simulink model "gm_uz_mpc_3ph"  (R2021a)
settings: Solver=FixedStepDiscrete  StartTime=0.0  StopTime=2000*t_ADC  RelTol=1e-3
undefined symbols (not defined in the file or in its folder): IB, id_ref, iq_ref, lambda_d, lambda_q, lambda_u, Ld_over_LB, Lq_over_LB, n_rpm, omegaB, p, psi_pm_over_psiB, Rs_over_ZB, t_ADC, t_clock, Ts_times_ZB_over_Ld, Ts_times_ZB_over_Lq, v_dc, VB
libraries: nesl_utility x19, simulink x18, fl_lib x15, ee_lib x7, hdlsllib x2, spsAlphaBetaZerotodq0Lib x1
(part 1 of 3)
settings Model: Creator=micha  LastModifiedBy=micha
settings SolverCC: AlgebraicLoopSolver=TrustRegion
settings DataIOCC: LimitDataPoints=on  SaveOutput=off  SaveTime=off
settings OptimizationCC: BlockReduction=off  ConditionallyExecuteInputs=off  DefaultParameterBehavior=Inlined  LifeSpan=inf
settings DebuggingCC: AlgebraicLoopMsg=error  InheritedTsInSrcMsg=none  SingleTaskRateTransMsg=error  AllowSymbolicDim=off  StrictBusMsg=ErrorOnBusTreatedAsVector  SFUnexpectedBacktrackingDiag=warning  SFNoUnconditionalDefaultTransitionDiag=warning  SFExecutionAtInitializationDiag=none  SFMachineParentedDataDiag=warning  ArithmeticOperatorsInVariantConditions=warning
settings HardwareCC: ProdBitPerPointer=32  ProdBitPerSizeT=32  ProdBitPerPtrDiffT=32  ProdLargestAtomicFloat=None  ProdIntDivRoundTo=Undefined  ProdEndianess=Unspecified  ProdWordSize=32  ProdHWDeviceType=ASIC/FPGA->ASIC/FPGA  ProdEqTarget=off
settings SFSimCC: SimUseLocalCustomCode=off  CustomCodeUndefinedFunction=UseInterfaceOnly
settings RTWCC: RTWUseLocalCustomCode=off
settings CodeAppCC: StateflowObjectComments=on
settings GRTTargetCC: TargetLangStandard=C89/C90 (ANSI)
settings ConfigComp: CovScope=ReferencedModels  CovMetricSettings=dw  CovSaveCumulativeToWorkspaceVar=on  CovSaveSingleToWorkspaceVar=on  CovExternalEMLEnable=off  CovSFcnEnable=off

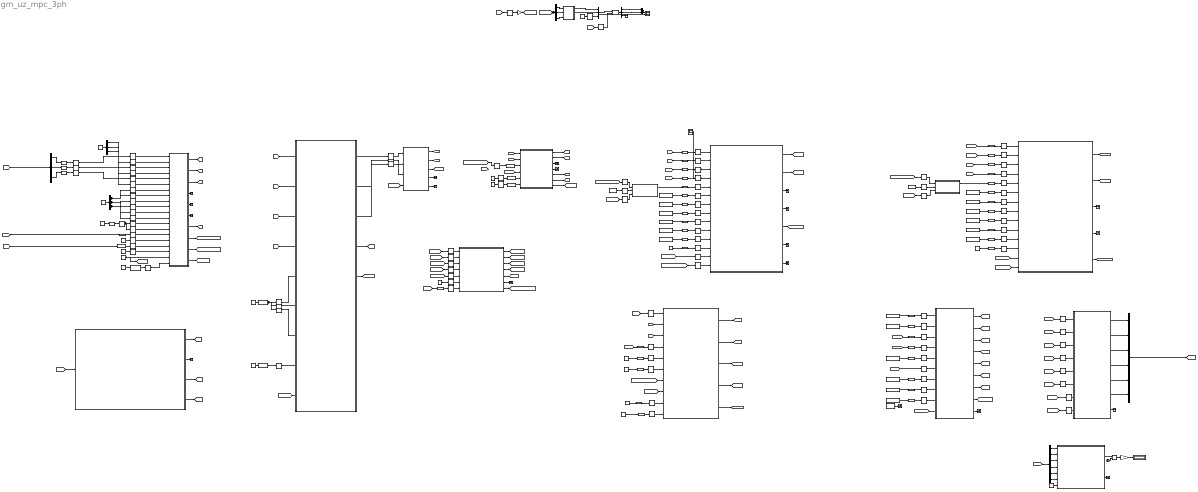
== system gm_uz_mpc_3ph ==
  note: 0=AXI 1=PL
  note: 1=real 0=debug
  note: delay compensation
  note: dynamic voltage LUT
  note: prediction model
  note: cost function
  note: gates enable
  note: average switching frequency calculation
  note: per unit conversion
  note: MPC state machine
  note: Clarke and Park transformation
  note: debug ip for input of constant measurement values
  note: inverter and motor
  Alpha-Beta-Zero to dq1 : spsAlphaBetaZerotodq0Lib/Alpha-Beta-Zero to dq0  Alignment=Aligned with phase A axis
      settings: SourceProductBaseCode=PS
  Clock : Clock
  Constant : Constant  Value=8  OutDataTypeStr=uint32  SampleTime=-1
  Constant1 : Constant  Value=p
  Constant10 : Constant  Value=psi_pm_over_psiB
  Constant{2,11,25,62} (4 alike) : Constant
  Constant12 : Constant  Value=0
  Constant13 : Constant  Value=p
  Constant14 : Constant  Value=psi_pm_over_psiB
  Constant15 : Constant  Value=Rs_over_ZB
  Constant17 : Constant  Value=Ts_times_ZB_over_Ld
  Constant18 : Constant  Value=Ts_times_ZB_over_Lq
  Constant21 : Constant  Value=Ld_over_LB
  Constant22 : Constant  Value=Lq_over_LB
  Constant26 : Constant  Value=v_dc
  Constant27 : Constant  Value=iq_ref/IB
  Constant3 : Constant  Value=Rs_over_ZB
  Constant30 : Constant  Value=0  OutDataTypeStr=uint32  SampleTime=-1
  Constant31 : Constant  Value=lambda_d
  Constant32 : Constant  Value=lambda_q
  Constant35 : Constant  Value=lambda_u
  Constant4 : Constant  Value=Ts_times_ZB_over_Ld
  Constant42 : Constant  Value=id_ref/IB
  Constant44 : Constant  Value=0.00008  SampleTime=-1
  Constant5 : Constant  Value=Ts_times_ZB_over_Lq
  Constant52 : Constant  Value=0
  Constant53 : Constant  Value=1/omegaB  OutDataTypeStr=fixdt(0,18,18)
  Constant54 : Constant  Value=1/omegaB  OutDataTypeStr=fixdt(0,18,18)
  Constant55 : Constant  Value=0  OutDataTypeStr=fixdt(1,24,11)  SampleTime=-1
  Constant56 : Constant  Value=1/IB
  Constant57 : Constant  Value=1/VB
  Constant58 : Constant  Value=63
  Constant59 : Constant  OutDataTypeStr=boolean  SampleTime=-1
  Constant6 : Constant  Value=[0 0 0]  OutDataTypeStr=fixdt(1,27,15)  SampleTime=-1
  Constant60 : Constant  Value=[1 2 3]  OutDataTypeStr=fixdt(1,27,15)  SampleTime=-1
  Constant61 : Constant  Value=0  OutDataTypeStr=fixdt(1,27,20)  SampleTime=-1
  Constant63 : Constant  Value=0.15
  Constant8 : Constant  Value=Ld_over_LB
  Constant9 : Constant  Value=Lq_over_LB
  Data Type Conversion1 : DataTypeConversion  OutDataTypeStr=boolean
  Data Type Conversion{2,6,10..11,13,65..66} (7 alike) : DataTypeConversion  OutDataTypeStr=fixdt_type_polepairs
  Data Type Conversion{12,14..15,18..22,25..28} (12 alike) : DataTypeConversion  OutDataTypeStr=fixdt_type_constants
  Data Type Conversion29 : DataTypeConversion  OutDataTypeStr=fixdt_type_speed
  Data Type Conversion30 : DataTypeConversion  OutDataTypeStr=fixdt_type_speed
  Data Type Conversion32 : DataTypeConversion  OutDataTypeStr=fixdt(0,18,18)
  Data Type Conversion33 : DataTypeConversion  OutDataTypeStr=fixdt(0,18,18)
  Data Type Conversion{34..36,68} (4 alike) : DataTypeConversion  OutDataTypeStr=fixdt(1,27,15)
  Data Type Conversion37 : DataTypeConversion  OutDataTypeStr=fixdt(1,27,20)
  Data Type Conversion39 : DataTypeConversion  OutDataTypeStr=fixdt(1,18,14)
  Data Type Conversion{4..5,44..45,52..53} (6 alike) : DataTypeConversion  OutDataTypeStr=fixdt_type_dq_currents
  Data Type Conversion{7..8,48..49} (4 alike) : DataTypeConversion  OutDataTypeStr=fixdt_type_dqxy_voltages
  Data Type Conversion54 : DataTypeConversion  OutDataTypeStr=fixdt_type_max_current
  Data Type Conversion57 : DataTypeConversion  OutDataTypeStr=fixdt_type_xy_currents
  Data Type Conversion58 : DataTypeConversion  OutDataTypeStr=fixdt_type_xy_currents
  Data Type Conversion59 : DataTypeConversion  OutDataTypeStr=fixdt(1,18,14)
  Data Type Conversion60 : DataTypeConversion  OutDataTypeStr=fixdt_type_lambda
  Data Type Conversion61 : DataTypeConversion  OutDataTypeStr=fixdt_type_lambda
  Data Type Conversion64 : DataTypeConversion  OutDataTypeStr=fixdt_type_lambda
  Data Type Conversion69 : DataTypeConversion  OutDataTypeStr=fixdt(1,24,11)
  Data Type Conversion70 : DataTypeConversion  OutDataTypeStr=fixdt(1,18,15)
  Data Type Conversion9 : DataTypeConversion  OutDataTypeStr=fixdt(1,27,20)
  Demux{,1,4..6} (5 alike) : Demux  Outputs=3
  Demux2 : Demux  Outputs=6
  Display : Display
  Divide : Product  Inputs=*/
  Gain : Gain  Gain=1/IB
  Gain19 : Gain  Gain=1/(6*2)
  Mux : Mux  Inputs=2
  Mux2 : Mux  Inputs=6
  Mux5 : Mux  Inputs=3
  Pulse Generator2 : DiscretePulseGenerator  PulseType=Time based  Period=t_ADC  PulseWidth=5
  Rate Transition : RateTransition  OutPortSampleTime=t_ADC
  Rate Transition{1..4,6..7,9..10,12..13,15,17..21,23,25,28..33,35,38..43,45..46,50,53..54,57..58,60..62,65..67,69..70,73..74,77..82,85..86,91..96,100..107,111..128,130} (89 alike) : RateTransition  OutPortSampleTime=t_clock
  Rate Transition{11,55,68,75..76,129} (6 alike) : RateTransition  InitialCondition=1  OutPortSampleTime=t_clock
  Rate Transition131 : RateTransition  OutPortSampleTime=t_ADC
  Rate Transition132 : RateTransition  OutPortSampleTime=t_ADC
  Scope : Scope  NumInputPorts=2
  Scope3 : Scope  NumInputPorts=2
  Terminator{,2..3,8..14,17..20,23..28} (20 alike) : Terminator
  clarke : MATLAB Function  TreatAsAtomicUnit=on
  cost_opt : Subsystem  TreatAsAtomicUnit=on
  counter_f_sw_3ph : Subsystem  TreatAsAtomicUnit=on
  ctrl_state_machine : Subsystem  TreatAsAtomicUnit=on
  delay_comp : Subsystem  TreatAsAtomicUnit=on
  inverter_machine : Subsystem
  mpc_enable : Subsystem  TreatAsAtomicUnit=on
  prediction : Subsystem  TreatAsAtomicUnit=on
  pu_omega_m : Subsystem  TreatAsAtomicUnit=on
  pu_omega_m1 : Subsystem
  pu_voltages_vsd : Subsystem  TreatAsAtomicUnit=on
  uz_clarke : Subsystem  TreatAsAtomicUnit=on
  uz_debug_switch_measurements : Subsystem  TreatAsAtomicUnit=on
  uz_park_transformation : Subsystem  TreatAsAtomicUnit=on
  uz_pu_conversion : Subsystem  TreatAsAtomicUnit=on
  wires:
  Demux1/3 -> Rate Transition121/1, Rate Transition122/1
  Demux1/2 -> Rate Transition120/1, Rate Transition119/1
  Demux1/1 -> Rate Transition117/1, Rate Transition118/1
  Constant6/1 -> Demux1/1
  Constant44/1 -> Terminator/1
  uz_pu_conversion/4(out3) -> [v_dc_pu]
  uz_debug_switch_measurements/6(out5) -> Terminator28/1
  uz_debug_switch_measurements/5(out4) -> Terminator27/1
  uz_debug_switch_measurements/4(out3) -> Terminator26/1
  [debug_ip_done] -> uz_pu_conversion/9(adc_valid_trigger)
  uz_debug_switch_measurements/10(debug_ip_done) -> [debug_ip_done]
  [v_dc] -> uz_pu_conversion/4(in3)
  [i_c1] -> uz_pu_conversion/3(in2)
  [i_b1] -> uz_pu_conversion/2(in1)
  [i_a1] -> uz_pu_conversion/1(in0)
  uz_debug_switch_measurements/3(out2) -> [i_c1]
  uz_debug_switch_measurements/7(out6) -> [v_dc]
  uz_debug_switch_measurements/2(out1) -> [i_b1]
  uz_debug_switch_measurements/1(out0) -> [i_a1]
  Mux/1 -> Scope/1
  Rate Transition132/1 -> Alpha-Beta-Zero to dq1/2
  Rate Transition131/1 -> Mux5/3
  Demux4/2 -> Mux/2  "iq"
  Demux4/1 -> Mux/1  "id"
  Rate Transition/1 -> Gain/1
  [pu_conv_valid] -> uz_clarke/4(pu_conv_valid)
  mpc_enable/7(enb_mpc_done) -> Terminator23/1
  [G1] -> Rate Transition96/1
  [G2] -> Rate Transition93/1
  [G3] -> Rate Transition94/1
  [G4] -> Rate Transition91/1
  [G5] -> Rate Transition92/1
  cost_opt/3(G1) -> [G1]
  cost_opt/4(G2) -> [G2]
  cost_opt/5(G3) -> [G3]
  cost_opt/6(G4) -> [G4]
  cost_opt/7(G5) -> [G5]
  [G0] -> Rate Transition95/1
  cost_opt/2(G0) -> [G0]
  prediction/4(iq_pred_pu_AXI) -> Terminator20/1
  prediction/3(id_pred_pu_AXI) -> Terminator19/1
  delay_comp/6(Rs_over_ZB) -> Terminator17/1
  delay_comp/7(Ts_times_ZB_over_Ld) -> Terminator18/1
  delay_comp/4(iq_delay_pu_AXI) -> Terminator14/1
  delay_comp/3(id_delay_pu_AXI) -> Terminator13/1
  ctrl_state_machine/6(trigger_state_machine_finished) -> Terminator12/1
  ctrl_state_machine/4(trigger_optimization) -> [trigger_optimization]
  [trigger_optimization] -> cost_opt/10(trigger_optimization)
  ctrl_state_machine/3(trigger_prediction) -> [trigger_prediciton]
  [trigger_prediciton] -> prediction/13(trigger_prediction)
  ctrl_state_machine/2(trigger_delay_comp) -> [trigger_delay_comp]
  [trigger_delay_comp] -> Rate Transition7/1
  uz_clarke/3(clarke_done) -> [clarke_done]
  [clarke_done] -> uz_park_transformation/4(trigger)
  [beta] -> uz_park_transformation/2(u2)
  [alpha] -> uz_park_transformation/1(u1)
  uz_clarke/1(alpha) -> [alpha]
  uz_clarke/2(beta) -> [beta]
  [trigger_voltages] -> pu_voltages_vsd/8(trigger_voltages)
  ctrl_state_machine/1(trigger_voltages) -> [trigger_voltages]
  Constant63/1 -> Data Type Conversion70/1
  Data Type Conversion70/1 -> Rate Transition130/1
  Rate Transition130/1 -> pu_voltages_vsd/9(v_DC_pu_AXI)
  Rate Transition129/1 -> pu_voltages_vsd/10(v_dc_select_AXI)
  Constant62/1 -> Data Type Conversion66/1
  Data Type Conversion66/1 -> Rate Transition129/1
  Demux6/1 -> Rate Transition111/1
  Demux6/2 -> Rate Transition113/1
  Demux6/3 -> Rate Transition116/1
  Constant60/1 -> Demux6/1
  uz_debug_switch_measurements/9(out8) -> [theta_el_from_debug_switch]
  Rate Transition128/1 -> uz_debug_switch_measurements/18(in0_AXI8)
  Constant61/1 -> Rate Transition128/1
  Rate Transition127/1 -> uz_debug_switch_measurements/17(in8)
  Data Type Conversion37/1 -> Rate Transition127/1
  [theta_el] -> Data Type Conversion37/1
  Constant55/1 -> Rate Transition126/1
  Data Type Conversion69/1 -> Rate Transition125/1
  uz_debug_switch_measurements/8(out7) -> [omega_m_from_debug_switch]
  [omega_m] -> Data Type Conversion69/1
  Rate Transition126/1 -> uz_debug_switch_measurements/16(in0_AXI7)
  Rate Transition125/1 -> uz_debug_switch_measurements/15(in7)
  Rate Transition124/1 -> uz_debug_switch_measurements/14(in0_AXI6)
  Rate Transition123/1 -> uz_debug_switch_measurements/13(in6)
  Rate Transition122/1 -> uz_debug_switch_measurements/12(in0_AXI5)
  Rate Transition121/1 -> uz_debug_switch_measurements/11(in5)
  Rate Transition120/1 -> uz_debug_switch_measurements/10(in0_AXI4)
  Rate Transition119/1 -> uz_debug_switch_measurements/9(in4)
  Rate Transition118/1 -> uz_debug_switch_measurements/8(in0_AXI3)
  Rate Transition117/1 -> uz_debug_switch_measurements/7(in3)
  Rate Transition116/1 -> uz_debug_switch_measurements/6(in0_AXI2)
  Rate Transition115/1 -> uz_debug_switch_measurements/3(in1)
  Rate Transition114/1 -> uz_debug_switch_measurements/5(in2)
  Rate Transition113/1 -> uz_debug_switch_measurements/4(in0_AXI1)
  Rate Transition112/1 -> uz_debug_switch_measurements/1(in0)
  Rate Transition111/1 -> uz_debug_switch_measurements/2(in0_AXI)
  Constant59/1 -> uz_debug_switch_measurements/19(real_or_debug_AXI), [debug_enb]
  Rate Transition10/1 -> uz_debug_switch_measurements/20(adc_valid_trigger)
  Rate Transition103/1 -> Rate Transition123/1, Rate Transition124/1
  Rate Transition100/1 -> Rate Transition114/1
  Rate Transition101/1 -> Rate Transition115/1
  Rate Transition102/1 -> Rate Transition112/1
  uz_pu_conversion/3(out2) -> Rate Transition33/1
  uz_pu_conversion/2(out1) -> Rate Transition32/1
  uz_pu_conversion/1(out0) -> Rate Transition35/1
  Constant58/1 -> Data Type Conversion65/1
  Data Type Conversion68/1 -> Rate Transition103/1
  Data Type Conversion36/1 -> Rate Transition100/1
  Data Type Conversion35/1 -> Rate Transition101/1
  Data Type Conversion34/1 -> Rate Transition102/1
  Data Type Conversion33/1 -> Rate Transition106/1, Rate Transition104/1, Rate Transition105/1
  Data Type Conversion32/1 -> Rate Transition107/1
  Constant57/1 -> Data Type Conversion32/1
  Constant56/1 -> Data Type Conversion33/1
  Rate Transition107/1 -> uz_pu_conversion/8(AXI_pu_conv_in3)
  Rate Transition104/1 -> uz_pu_conversion/7(AXI_pu_conv_in2)
  Rate Transition105/1 -> uz_pu_conversion/6(AXI_pu_conv_in1)
  Rate Transition106/1 -> uz_pu_conversion/5(AXI_pu_conv_in0)
  Constant26/1 -> Data Type Conversion68/1
  Rate Transition96/1 -> mpc_enable/2(G1)
  Rate Transition95/1 -> mpc_enable/1(G0)
  Rate Transition93/1 -> mpc_enable/3(G2)
  Rate Transition94/1 -> mpc_enable/4(G3)
  Rate Transition92/1 -> mpc_enable/6(G5)
  Rate Transition91/1 -> mpc_enable/5(G4)
  Rate Transition86/1 -> mpc_enable/8(adc_valid_trigger)
  Rate Transition85/1 -> mpc_enable/7(AXI_mpc_enb)
  [debug_enb] -> Rate Transition85/1
  [pu_conv_valid] -> Rate Transition86/1
  mpc_enable/4(out_G3) -> Mux2/4
  mpc_enable/6(out_G5) -> Mux2/6
  mpc_enable/3(out_G2) -> Mux2/3
  mpc_enable/5(out_G4) -> Mux2/5
  mpc_enable/2(out_G1) -> Mux2/2
  mpc_enable/1(out_G0) -> Mux2/1
  Mux2/1 -> [opt_gates]
  [omega_m_from_debug_switch] -> Rate Transition82/1
  Rate Transition81/1 -> pu_omega_m1/2(AXI_pu_conv_in)
  Constant54/1 -> Rate Transition81/1
  [pu_conv_valid] -> Rate Transition80/1
  Rate Transition82/1 -> pu_omega_m1/1(in1)
  Rate Transition80/1 -> pu_omega_m1/3(adc_valid_trigger)
  Rate Transition79/1 -> pu_omega_m/1(in1)
  Rate Transition78/1 -> pu_omega_m/2(AXI_pu_conv_in)
  Rate Transition77/1 -> pu_omega_m/3(adc_valid_trigger)
  Constant53/1 -> Rate Transition78/1
  [pu_conv_valid] -> Rate Transition77/1
  [omega_m_from_debug_switch] -> Rate Transition79/1
  Demux4/3 -> Terminator11/1
  clarke/2(beta) -> Mux5/2  "beta"
  Alpha-Beta-Zero to dq1/1 -> Demux4/1
  Mux5/1 -> Alpha-Beta-Zero to dq1/1
  clarke/1(alpha) -> Mux5/1  "alpha"
  [theta_el] -> Rate Transition132/1
  Constant52/1 -> Rate Transition131/1
  Gain/1 -> [pu_phase_currents]
  [i_ph] -> Rate Transition/1
  Demux5/1 -> clarke/1(a1)
  [pu_phase_currents] -> Demux5/1, Scope/2
  Demux5/3 -> clarke/3(c1)
  Demux5/2 -> clarke/2(b1)
  Rate Transition7/1 -> delay_comp/13(trigger_delay_comp)
  Rate Transition6/1 -> delay_comp/14(trigger_park_done)
  [trigger_park_done_statemachine] -> Rate Transition6/1
  ctrl_state_machine/7(trigger_park_done_statemachine) -> [trigger_park_done_statemachine]
  delay_comp/2(iq_delay_pu) -> [iq_delay_pu]
  delay_comp/1(id_delay_pu) -> [id_delay_pu]  "id_delay"
  [opt_gates] -> inverter_machine/1(In1)
  Rate Transition41/1 -> delay_comp/1(id_pu)  "id_measured"
  ctrl_state_machine/5(index) -> [index]
  [trigger_park_done_statemachine] -> pu_voltages_vsd/7(trigger_park_done)
  [delay_comp_done] -> prediction/14(trigger_delay_comp_done)
  [trigger_park_done] -> Rate Transition58/1
  Rate Transition39/1 -> delay_comp/7(Ts_times_ZB_over_Ld_AXI)
  Rate Transition62/1 -> cost_opt/5(max_current_pu_AXI)
  Data Type Conversion29/1 -> Rate Transition43/1
  Rate Transition45/1 -> delay_comp/2(iq_pu)
  pu_omega_m/1(out1) -> Data Type Conversion29/1
  Data Type Conversion7/1 -> Rate Transition67/1
  Data Type Conversion25/1 -> Rate Transition29/1
  Rate Transition30/1 -> delay_comp/10(Lq_over_LB_AXI)
  Constant31/1 -> Data Type Conversion60/1
  Rate Transition42/1 -> delay_comp/8(Ts_times_ZB_over_Lq_AXI)
  Data Type Conversion26/1 -> Rate Transition30/1
  Constant3/1 -> Data Type Conversion20/1
  Data Type Conversion5/1 -> Rate Transition45/1
  Demux2/5 -> counter_f_sw_3ph/5(ss_in_4)
  Rate Transition25/1 -> delay_comp/6(Rs_over_ZB_AXI)
  prediction/1(id_pred_pu) -> [id_pred_pu]
  Data Type Conversion2/1 -> Rate Transition11/1
  [vq_pu] -> Data Type Conversion49/1
  Data Type Conversion54/1 -> Rate Transition62/1
  counter_f_sw_3ph/2(switchNumb) -> Terminator24/1
  Data Type Conversion53/1 -> Rate Transition60/1
  Rate Transition66/1 -> cost_opt/2(iq_ref_pu_AXI)
  [id_pu] -> Data Type Conversion4/1
  [id_delay_pu] -> Data Type Conversion44/1
  Data Type Conversion8/1 -> Rate Transition74/1
  Data Type Conversion49/1 -> Rate Transition54/1
  Data Type Conversion52/1 -> Rate Transition57/1
  Rate Transition31/1 -> delay_comp/11(psi_pm_over_psiB_AXI)
  [id_pred_pu] -> Data Type Conversion52/1
  Data Type Conversion44/1 -> Rate Transition28/1
  Rate Transition55/1 -> pu_voltages_vsd/6(index_AXI)
  Rate Transition28/1 -> prediction/1(id_delay_pu)
  [iq_pred_pu] -> Data Type Conversion53/1
  Data Type Conversion6/1 -> Rate Transition75/1
  Constant27/1 -> Data Type Conversion58/1
  Rate Transition23/1 -> prediction/5(omega_m_pu)
  Rate Transition57/1 -> cost_opt/3(id_pred_pu)
  Divide/1 -> Gain19/1
  Rate Transition65/1 -> cost_opt/1(id_ref_pu_AXI)
  Constant5/1 -> Data Type Conversion22/1
  Constant42/1 -> Data Type Conversion57/1
  Data Type Conversion60/1 -> Rate Transition69/1
  Rate Transition76/1 -> ctrl_state_machine/7(last_opt_index)
  Data Type Conversion22/1 -> Rate Transition42/1
  Data Type Conversion61/1 -> Rate Transition70/1
  Demux2/4 -> counter_f_sw_3ph/4(ss_in_3)
  Data Type Conversion64/1 -> Rate Transition73/1
  Rate Transition73/1 -> cost_opt/9(lambda_u_AXI)
  Constant4/1 -> Data Type Conversion21/1
  Constant35/1 -> Data Type Conversion64/1
  cost_opt/8(optimization_done) -> [optimization_done]  "optimization done"
  Rate Transition60/1 -> cost_opt/4(iq_pred_pu)
  Data Type Conversion20/1 -> Rate Transition25/1
  [iq_pu] -> Data Type Conversion5/1
  Rate Transition13/1 -> prediction/6(Rs_over_ZB_AXI)
  cost_opt/1(opt_index) -> [opt_index]  "result"
  Rate Transition53/1 -> prediction/3(vd_pu)
  prediction/5(prediction_done) -> [prediction_done]
  Constant1/1 -> Data Type Conversion13/1
  [vd_pu] -> Data Type Conversion48/1
  Constant10/1 -> Data Type Conversion28/1
  Data Type Conversion11/1 -> Rate Transition12/1
  Rate Transition43/1 -> delay_comp/5(omega_m_pu)
  [opt_index] -> Data Type Conversion10/1
  Data Type Conversion13/1 -> Rate Transition15/1
  Rate Transition17/1 -> prediction/9(Ld_over_LB_AXI)
  Rate Transition29/1 -> delay_comp/9(Ld_over_LB_AXI)
  Rate Transition20/1 -> prediction/7(Ts_times_ZB_over_Ld_AXI)
  Rate Transition12/1 -> prediction/12(polepairs_AXI)
  Data Type Conversion48/1 -> Rate Transition53/1
  Data Type Conversion10/1 -> Rate Transition76/1
  Data Type Conversion19/1 -> Rate Transition18/1
  Constant11/1 -> Data Type Conversion54/1
  Constant32/1 -> Data Type Conversion61/1
  [vd_pu] -> Data Type Conversion7/1
  Data Type Conversion27/1 -> Rate Transition19/1
  [index] -> Rate Transition68/1
  pu_voltages_vsd/4(pu_vq_AXI) -> [vq_pu_AXI]
  Rate Transition70/1 -> cost_opt/8(lambda_q_AXI)
  [sin] -> pu_voltages_vsd/2(sin_angle)
  Rate Transition54/1 -> prediction/4(vq_pu)
  Rate Transition69/1 -> cost_opt/7(lambda_d_AXI)
  Data Type Conversion28/1 -> Rate Transition31/1
  Gain19/1 -> Display/1
  Demux2/6 -> counter_f_sw_3ph/6(ss_in_5)
  Rate Transition11/1 -> pu_voltages_vsd/5(index_select_AXI)
  Data Type Conversion57/1 -> Rate Transition65/1
  Rate Transition68/1 -> cost_opt/6(index)
  Rate Transition18/1 -> prediction/10(Lq_over_LB_AXI)
  Demux2/1 -> counter_f_sw_3ph/1(ss_in_0)
  [index] -> Data Type Conversion6/1
  Data Type Conversion4/1 -> Rate Transition41/1
  prediction/2(iq_pred_pu) -> [iq_pred_pu]
  Data Type Conversion58/1 -> Rate Transition66/1
  Demux2/3 -> counter_f_sw_3ph/3(ss_in_2)
  Clock/1 -> Divide/2
  Constant9/1 -> Data Type Conversion26/1
  Demux2/2 -> counter_f_sw_3ph/2(ss_in_1)
  Data Type Conversion30/1 -> Rate Transition23/1
  [opt_gates] -> Demux2/1
  Rate Transition67/1 -> delay_comp/3(vd_pu), Scope3/1
  cost_opt/9(costs) -> Terminator10/1
  Rate Transition50/1 -> prediction/2(iq_delay_pu)
  pu_voltages_vsd/3(pu_vd_AXI) -> [vd_pu_AXI]
  Constant17/1 -> Data Type Conversion14/1
  Rate Transition21/1 -> prediction/8(Ts_times_ZB_over_Lq_AXI)
  counter_f_sw_3ph/1(switchNumb_AXI) -> Divide/1
  Data Type Conversion15/1 -> Rate Transition21/1
  [iq_delay_pu] -> Data Type Conversion45/1
  Constant30/1 -> counter_f_sw_3ph/7(bResetAXI)
  Rate Transition46/1 -> pu_voltages_vsd/1(v_DC_pu)
  [cos] -> pu_voltages_vsd/3(cos_angle)
  Constant2/1 -> Data Type Conversion2/1
  Data Type Conversion45/1 -> Rate Transition50/1
  pu_voltages_vsd/2(pu_vq) -> [vq_pu]
  Data Type Conversion18/1 -> Rate Transition17/1
  delay_comp/5(delay_comp_done) -> [delay_comp_done]
  [vq_pu] -> Data Type Conversion8/1
  Rate Transition75/1 -> pu_voltages_vsd/4(index)
  Constant8/1 -> Data Type Conversion25/1
  Data Type Conversion21/1 -> Rate Transition39/1
  pu_omega_m1/1(out1) -> Data Type Conversion30/1
  Constant18/1 -> Data Type Conversion15/1
  Constant21/1 -> Data Type Conversion18/1
  Constant15/1 -> Data Type Conversion12/1
  Rate Transition19/1 -> prediction/11(psi_pm_over_psiB_AXI)
  Data Type Conversion14/1 -> Rate Transition20/1
  Rate Transition74/1 -> delay_comp/4(vq_pu), Scope3/2
  Constant22/1 -> Data Type Conversion19/1
  [v_dc_pu] -> Rate Transition46/1
  pu_voltages_vsd/1(pu_vd) -> [vd_pu]
  pu_voltages_vsd/5(voltages_done) -> [voltages_done]  "calc_done"
  Rate Transition15/1 -> delay_comp/12(polepairs_AXI)
  Data Type Conversion65/1 -> Rate Transition55/1
  Data Type Conversion12/1 -> Rate Transition13/1
  Constant14/1 -> Data Type Conversion27/1
  Constant13/1 -> Data Type Conversion11/1
  uz_park_transformation/4(y2_AXI) -> Terminator9/1
  [theta_el_from_debug_switch] -> Rate Transition38/1
  uz_park_transformation/6(cos) -> [cos]
  Pulse Generator2/1 -> Data Type Conversion1/1
  Data Type Conversion1/1 -> Rate Transition10/1
  uz_pu_conversion/5(pu_conv_done) -> [pu_conv_valid]
  Demux/1 -> Data Type Conversion34/1
  Rate Transition32/1 -> uz_clarke/2(b1)
  Demux/3 -> Data Type Conversion36/1
  Constant25/1 -> Rate Transition40/1
  Rate Transition35/1 -> uz_clarke/1(a1)
  [i_ph] -> Demux/1
  inverter_machine/1(i_ph) -> [i_ph]
  uz_park_transformation/5(sin) -> [sin]
  uz_clarke/5(beta_AXI) -> Terminator3/1
  inverter_machine/2(i_dc) -> Terminator25/1
  inverter_machine/3(theta_el) -> [theta_el]
  inverter_machine/4(omega_m) -> [omega_m]
  uz_park_transformation/1(y1) -> [id_pu]  "id_pu"
  Rate Transition33/1 -> uz_clarke/3(c1)
  Demux/2 -> Data Type Conversion35/1
  Constant12/1 -> Rate Transition61/1
  Rate Transition40/1 -> Data Type Conversion39/1
  Rate Transition61/1 -> Data Type Conversion59/1
  Data Type Conversion59/1 -> uz_park_transformation/6(offset_angle_el_AXI)
  uz_park_transformation/2(y2) -> [iq_pu]  "iq_pu"
  Data Type Conversion9/1 -> uz_park_transformation/3(angle_el)
  uz_clarke/4(alpha_AXI) -> Terminator2/1
  uz_park_transformation/3(y1_AXI) -> Terminator8/1
  Data Type Conversion39/1 -> uz_park_transformation/5(factor_angle_el_AXI)
  Rate Transition38/1 -> Data Type Conversion9/1
  uz_park_transformation/7(park_done) -> [trigger_park_done]  "calc_done"
  Constant/1 -> Rate Transition9/1
  Rate Transition9/1 -> ctrl_state_machine/6(AXI_no_of_iterations)  "opt_done"
  Rate Transition4/1 -> ctrl_state_machine/5(trigger_optimization_done)  "opt_done"
  Rate Transition3/1 -> ctrl_state_machine/4(trigger_prediction_done)  "pred_done"
  Rate Transition2/1 -> ctrl_state_machine/3(trigger_delay_comp_done)  "delay_done"
  Rate Transition1/1 -> ctrl_state_machine/2(trigger_voltages_done)  "volts_done"
  Rate Transition58/1 -> ctrl_state_machine/1(trigger_start_state_machine)  "park_done"
  [voltages_done] -> Rate Transition1/1
  [delay_comp_done] -> Rate Transition2/1
  [prediction_done] -> Rate Transition3/1
  [optimization_done] -> Rate Transition4/1

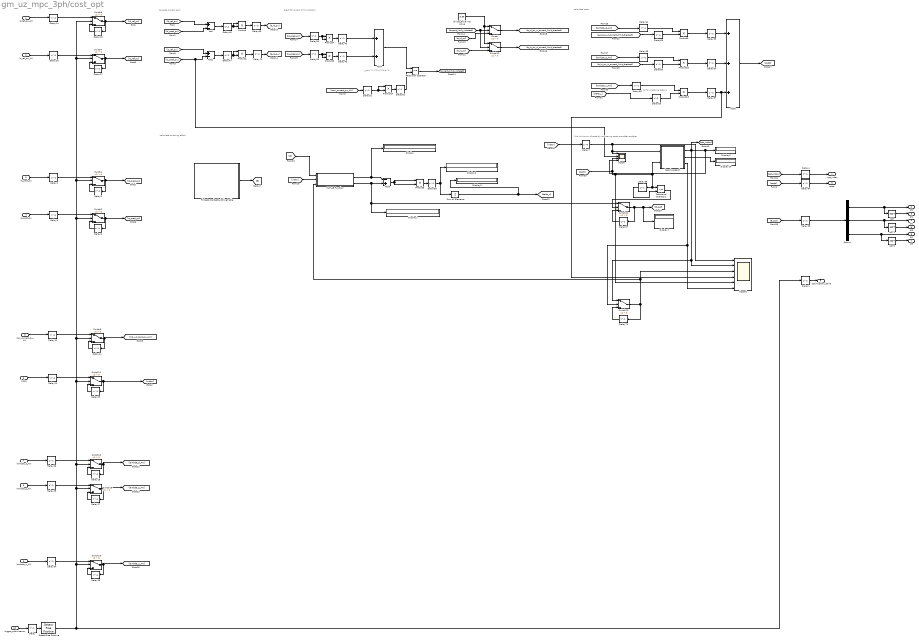
== system gm_uz_mpc_3ph/cost_opt ==
  note: squared current error
  note: check for current limit violation
  note: calculate switching effort
  note: calculate costs
  note: find minimum of costs by comparing costs one after another
  note: i_max^2 <= id^2+iq^2
  note: z-2 for matching delays
  id_ref_pu_AXI : Inport
  iq_ref_pu_AXI : Inport  Port=2
  id_pred_pu : Inport  Port=3
  iq_pred_pu : Inport  Port=4
  max_current_pu_AXI : Inport  Port=5
  index : Inport  Port=6
  lambda_d_AXI : Inport  Port=7
  lambda_q_AXI : Inport  Port=8
  lambda_u_AXI : Inport  Port=9
  trigger_optimization : Inport  Port=10
  Add : Sum  Inputs=+-
  Add1 : Sum  Inputs=+-
  Add4 : Sum  AccumDataTypeStr=fixdt_type_squared_current_error
  Add5 : Sum  Inputs=-+
  Add6 : Sum  Inputs=+++  AccumDataTypeStr=fixdt_type_delta_u_costs
  Delay{,1..6,11..12,14..17,25..28,33..34,36,38..39,42..43,46..47,51..54,57..60,64..65,68..70,94} (40 alike) : Delay  DelayLength=1
  Delay23 : Delay  DelayLength=1  InitialCondition=1
  Delay24 : Delay  DelayLength=1  InitialCondition=1
  Delay35 : Delay  DelayLength=1  InitialCondition=4.99
  Delay37 : Delay  DelayLength=1  InitialCondition=0
  Delay63 : Delay
  Delay7 : Delay  DelayLength=4  InitialCondition=1
  Delay73 : Delay  DelayLength=1  InitialCondition=1
  Demux : Demux  Outputs=3
  Detect Rise Positive : simulink/Logic and Bit Operations/Detect Rise Positive  vinit=0  OutDataTypeStr=boolean
  Display{,1..3,6..7,10} (7 alike) : Display
  FiniteControlSetSwitchingTable : MATLAB Function  TreatAsAtomicUnit=on
  MATLAB Function : MATLAB Function  TreatAsAtomicUnit=on
  NOT : Logic  Operator=NOT  IconShape=distinctive  AllPortsSameDT=off  OutDataTypeStr=boolean
  NOT1 : Logic  Operator=NOT  IconShape=distinctive  AllPortsSameDT=off  OutDataTypeStr=boolean
  NOT2 : Logic  Operator=NOT  IconShape=distinctive  AllPortsSameDT=off  OutDataTypeStr=boolean
  Product{,1,4..5,9..10,14} (7 alike) : Product  OutDataTypeStr=fixdt_type_squared_current_error
  Product13 : Product  OutDataTypeStr=fixdt_type_delta_u_costs
  Product8 : Product  OutDataTypeStr=uint16
  Relational Operator : RelationalOperator  OutDataTypeStr=boolean  RndMeth=Simplest
  Relational Operator1 : RelationalOperator  Operator=<=  OutDataTypeStr=boolean  RndMeth=Simplest
  Scope : Scope  NumInputPorts=4
  Scope1 : Scope  NumInputPorts=6
  Sum of Elements : Sum  Inputs=+  AccumDataTypeStr=uint16
  Switch{,1..2,5..7,11..12,15..16,19..21} (13 alike) : Switch  Criteria=u2 > Threshold
  iterativesearch : MATLAB Function  TreatAsAtomicUnit=on
  sfix18_En15 max value : Constant  Value=3.99  OutDataTypeStr=fixdt(1,18,15)  SampleTime=-1
  opt_index : Outport  VectorParamsAs1DForOutWhenUnconnected=off
  G0 : Outport  Port=2  VectorParamsAs1DForOutWhenUnconnected=off
  G1 : Outport  Port=3  VectorParamsAs1DForOutWhenUnconnected=off
  G2 : Outport  Port=4  VectorParamsAs1DForOutWhenUnconnected=off
  G3 : Outport  Port=5  VectorParamsAs1DForOutWhenUnconnected=off
  G4 : Outport  Port=6  VectorParamsAs1DForOutWhenUnconnected=off
  G5 : Outport  Port=7  VectorParamsAs1DForOutWhenUnconnected=off
  optimization_done : Outport  Port=8  VectorParamsAs1DForOutWhenUnconnected=off
  costs : Outport  Port=9  VectorParamsAs1DForOutWhenUnconnected=off
  wires:
  Delay7/1 -> Scope/1, iterativesearch/1(index), Scope1/1
  Delay63/1 -> Product13/2  "dU"
  [index] -> MATLAB Function/2(index)
  iterativesearch/2(min_costs) -> Display10/1
  iterativesearch/3(opt_done) -> Switch20/2, Scope1/6
  iterativesearch/1(opt_idx) -> [opt_index], Display6/1, Scope/4, Switch20/1, Scope1/2  "opt_idx"
  Delay73/1 -> Switch20/3
  MATLAB Function/2(G_prev) -> Add5/2, Switch21/1, Display1/1
  Switch20/1 -> Scope1/3, MATLAB Function/3(last_optim_index), Delay73/1  "last_opt_idx"
  Sum of Elements/1 -> Display3/1, [delta_u]
  Delay70/1 -> [e_iq_pu]
  Delay69/1 -> [e_id_pu]
  Delay68/1 -> Product13/1
  Delay65/1 -> Product10/1
  Delay64/1 -> Product9/1
  Delay60/1 -> Product10/2
  Delay59/1 -> Product9/2
  Delay58/1 -> Display2/1, Sum of Elements/1
  Delay57/1 -> Add6/3, Scope1/4  "dU"
  Delay54/1 -> Add6/2
  Delay53/1 -> Add6/1
  Delay52/1 -> Relational Operator/2
  Delay51/1 -> Product14/2, Product14/1
  Switch11/1 -> Delay23/1, [index]
  Delay47/1 -> Product1/2, Product1/1
  Delay46/1 -> Product/2, Product/1
  Delay43/1 -> Add4/2
  Delay42/1 -> Add4/1
  Delay39/1 -> Product5/1, Product5/2
  Delay36/1 -> Product4/1, Product4/2
  [G_opt] -> Delay38/1
  Relational Operator1/1 -> Switch21/2
  Delay35/1 -> Relational Operator1/2
  [index] -> Delay7/1  "idx"
  [costs] -> iterativesearch/2(cost), Relational Operator1/1, Delay35/1, Scope1/5, Scope/3  "costs"
  Detect Rise Positive/1 -> Delay1/1, Switch19/2, Switch16/2, Switch15/2, Switch11/2, Switch5/2, Switch7/2, Switch6/2, Switch1/2, Switch2/2
  Switch21/1 -> Delay37/1, [G_opt], Display7/1
  Delay37/1 -> Switch21/3
  Delay94/1 -> costs/1
  [costs] -> Delay94/1
  Product14/1 -> Delay52/1
  [max_current_pu_AXI] -> Delay51/1
  Switch/1 -> [e_id_pu_w_current_limit_checked]
  Switch12/1 -> [e_iq_pu_w_current_limit_checked]
  Relational Operator/1 -> [current_limit_violated]
  [iq_pred_pu] -> Delay39/1
  [id_pred_pu] -> Delay36/1
  Product5/1 -> Delay43/1
  Product4/1 -> Delay42/1
  Product/1 -> Delay69/1
  Product1/1 -> Delay70/1
  Add/1 -> Delay46/1
  Add1/1 -> Delay47/1
  [iq_ref_pu] -> Add1/1
  [iq_pred_pu] -> Add1/2, Scope/2
  [id_pred_pu] -> Add/2
  [id_ref_pu] -> Add/1
  [e_iq_pu_w_current_limit_checked] -> Delay60/1
  [e_id_pu_w_current_limit_checked] -> Delay59/1
  [delta_u] -> Delay63/1
  [lambda_u_AXI] -> Delay68/1
  [lambda_q_AXI] -> Delay65/1
  [lambda_d_AXI] -> Delay64/1
  Add6/1 -> [costs]
  Product13/1 -> Delay57/1
  Product10/1 -> Delay54/1
  Product9/1 -> Delay53/1
  MATLAB Function/1(G_next) -> Add5/1, Display/1
  Add5/1 -> Product8/2, Product8/1
  Product8/1 -> Delay58/1
  Demux/3 -> NOT2/1, G4/1
  Demux/2 -> NOT1/1, G2/1
  NOT1/1 -> G3/1
  NOT2/1 -> G5/1
  Demux/1 -> NOT/1, G0/1
  NOT/1 -> G1/1
  Add4/1 -> Relational Operator/1
  Delay38/1 -> Demux/1
  [opt_index] -> Delay4/1
  Delay34/1 -> Switch19/1
  lambda_u_AXI/1 -> Delay34/1
  Switch19/1 -> Delay33/1, [lambda_u_AXI]
  Delay33/1 -> Switch19/3
  Delay27/1 -> Switch16/3
  Switch16/1 -> Delay27/1, [lambda_q_AXI]
  Delay28/1 -> Switch16/1
  lambda_q_AXI/1 -> Delay28/1
  lambda_d_AXI/1 -> Delay26/1
  Switch15/1 -> Delay25/1, [lambda_d_AXI]
  Delay25/1 -> Switch15/3
  Delay26/1 -> Switch15/1
  [G] -> MATLAB Function/1(in)
  sfix18_En15 max value/1 -> Switch12/1, Switch/1
  [e_iq_pu] -> Switch12/3
  [current_limit_violated] -> Switch/2, Switch12/2
  [e_id_pu] -> Switch/3
  Delay23/1 -> Switch11/3
  index/1 -> Delay24/1
  Delay24/1 -> Switch11/1
  FiniteControlSetSwitchingTable/1(G) -> [G]
  Switch5/1 -> Delay11/1, [max_current_pu_AXI]
  Delay11/1 -> Switch5/3
  Delay12/1 -> Switch5/1
  max_current_pu_AXI/1 -> Delay12/1
  id_pred_pu/1 -> Delay2/1
  Delay3/1 -> Switch1/3
  Delay6/1 -> Switch2/3
  Switch2/1 -> Delay6/1, [iq_pred_pu]
  iq_pred_pu/1 -> Delay5/1
  Delay5/1 -> Switch2/1
  Delay2/1 -> Switch1/1
  Switch1/1 -> Delay3/1, [id_pred_pu]
  Delay14/1 -> Switch6/1
  Switch6/1 -> Delay15/1, [id_ref_pu]
  Delay15/1 -> Switch6/3
  Delay16/1 -> Switch7/1
  iq_ref_pu_AXI/1 -> Delay16/1
  Switch7/1 -> Delay17/1, [iq_ref_pu]
  id_ref_pu_AXI/1 -> Delay14/1
  Delay17/1 -> Switch7/3
  Delay4/1 -> opt_index/1
  Delay1/1 -> optimization_done/1
  Delay/1 -> Detect Rise Positive/1
  trigger_optimization/1 -> Delay/1

== system gm_uz_mpc_3ph/counter_f_sw_3ph ==
  note: 1 for one cycle if edge recognized
  ss_in_0 : Inport  OutDataTypeStr=boolean  PortDimensions=1  SampleTime=1e-08
  ss_in_1 : Inport  Port=2  OutDataTypeStr=boolean  PortDimensions=1  SampleTime=1e-08
  ss_in_2 : Inport  Port=3  OutDataTypeStr=boolean  PortDimensions=1  SampleTime=1e-08
  ss_in_3 : Inport  Port=4  OutDataTypeStr=boolean  PortDimensions=1  SampleTime=1e-08
  ss_in_4 : Inport  Port=5  OutDataTypeStr=boolean  PortDimensions=1  SampleTime=1e-08
  ss_in_5 : Inport  Port=6  OutDataTypeStr=boolean  PortDimensions=1  SampleTime=1e-08
  bResetAXI : Inport  Port=7  OutDataTypeStr=uint32  PortDimensions=1  SampleTime=1e-08
  Count_f_sw : Subsystem
  Detec_edge : Sum  Inputs=+-  AccumDataTypeStr=int8  OutDataTypeStr=int8  SampleTime=1e-08
  SS_Old : Delay  DelayLength=double(1)  InitialCondition=0  SampleTime=1e-08
  Saturation : Saturate  UpperLimit="fi(0,0,1,0,\"hex\",\"1\")"  LowerLimit="fi(0,0,1,0,\"hex\",\"0\")"  SampleTime=1e-08  OutDataTypeStr=fixdt(0, 1, 0)
  delay : Delay  DelayLength=double(1)  InitialCondition=0  SampleTime=1e-08
  dtc : DataTypeConversion  OutDataTypeStr=fixdt(0, 1, 0)  SampleTime=1e-08  SaturateOnIntegerOverflow=on
  mux : Mux  Inputs=6
  reset_old2 : Delay  DelayLength=double(1)  InitialCondition=0  SampleTime=1e-08
  reset_old_switch1 : Switch  Criteria=u2 ~= 0  Threshold=double(0)  OutDataTypeStr=uint32  SampleTime=1e-08
  switchNumb_AXI : Outport  SampleTime=1e-08  VectorParamsAs1DForOutWhenUnconnected=off
  switchNumb : Outport  Port=2  SampleTime=1e-08  VectorParamsAs1DForOutWhenUnconnected=off
  wires:
  ss_in_0/1 -> mux/1
  ss_in_1/1 -> mux/2
  ss_in_2/1 -> mux/3
  ss_in_3/1 -> mux/4
  ss_in_4/1 -> mux/5
  ss_in_5/1 -> mux/6
  bResetAXI/1 -> reset_old_switch1/1, Detec_edge/1
  Count_f_sw/1(switchNumbOut) -> delay/1, switchNumb_AXI/1, switchNumb/1
  Detec_edge/1 -> reset_old_switch1/2, dtc/1
  mux/1 -> SS_Old/1, Count_f_sw/3(ss_v)
  SS_Old/1 -> Count_f_sw/2(ss_v_old)
  Saturation/1 -> Count_f_sw/4(bReset)
  delay/1 -> Count_f_sw/1(switchNumb)
  reset_old2/1 -> reset_old_switch1/3, Detec_edge/2
  reset_old_switch1/1 -> reset_old2/1
  dtc/1 -> Saturation/1

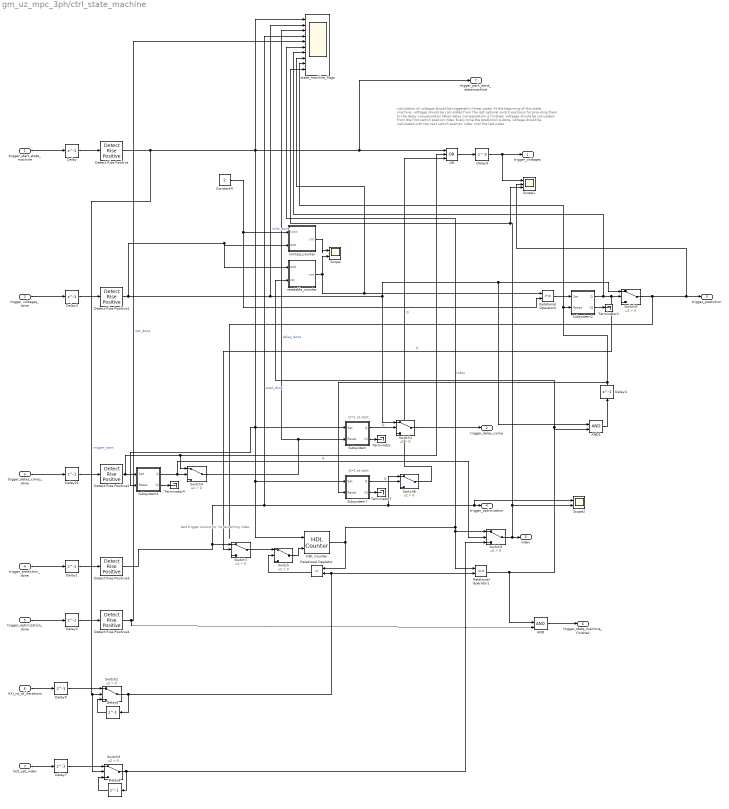
== system gm_uz_mpc_3ph/ctrl_state_machine ==
  note: Q=1 at start
  note: Q=1 at start
  note: calculation of voltages should be triggered in three cases:
      |
      | At the beginning of this state machine, voltages should be calculated from the last optimal switch positions for providing them to the delay compensation
      | When delay compensation is finished, voltages should be calculated from the first switch position index
      | Every time the prediciton is done, voltage should be calculated with the next switch position index until the last index
  note: test trigger source for incrementing index
  trigger_start_state_machine : Inport
  trigger_voltages_done : Inport  Port=2
  trigger_delay_comp_done : Inport  Port=3
  trigger_prediction_done : Inport  Port=4
  trigger_optimization_done : Inport  Port=5
  AXI_no_of_iterations : Inport  Port=6  OutDataTypeStr=uint32
  last_opt_index : Inport  Port=7  OutDataTypeStr=uint32
  AND : Logic  IconShape=distinctive  AllPortsSameDT=off  OutDataTypeStr=boolean
  AND1 : Logic  IconShape=distinctive  AllPortsSameDT=off  OutDataTypeStr=boolean
  Constant4 : Constant  Value=2  OutDataTypeStr=uint8  SampleTime=-1
  Delay{,1..8,21} (10 alike) : Delay  DelayLength=1
  Delay9 : Delay  DelayLength=3
  Detect Rise Positive{,1..4} (5 alike) : simulink/Logic and Bit Operations/Detect Rise Positive  vinit=0  OutDataTypeStr=boolean
  HDL Counter : hdlsllib/Sources/HDL Counter  CountType=Free running  CountInit=1  CountStep=1  CountMax=25  CountFromType=Initial value  CountFrom=1  CountResetPort=on  CountLoadPort=off  CountEnbPort=on  CountDirPort=off  CountHitOutputPort=off  CountDataType=Unsigned  CountWordLen=32  CountFracLen=0  CountSampTime=1
  OR : Logic  Operator=OR  Inputs=3  IconShape=distinctive  AllPortsSameDT=off  OutDataTypeStr=boolean
  Relational Operator : RelationalOperator  Operator=<  OutDataTypeStr=boolean  RndMeth=Simplest
  Relational Operator1 : RelationalOperator  Operator===  OutDataTypeStr=boolean  RndMeth=Simplest
  Relational Operator2 : RelationalOperator  OutDataTypeStr=boolean  RndMeth=Simplest
  Scope : Scope  NumInputPorts=2
  Scope1 : Scope  NumInputPorts=3
  Scope2 : Scope  NumInputPorts=2
  Subsystem : Subsystem
  Subsystem2 : Subsystem
  Subsystem4 : Subsystem
  Subsystem7 : Subsystem
  Switch{,1..5,7..9} (9 alike) : Switch  Criteria=u2 > Threshold
  Terminator{,2,4,7} (4 alike) : Terminator
  limited_counter : Subsystem
  resetable_counter : Subsystem
  state_machine_flags : Scope  NumInputPorts=10
  trigger_voltages : Outport  VectorParamsAs1DForOutWhenUnconnected=off
  trigger_delay_comp : Outport  Port=2  VectorParamsAs1DForOutWhenUnconnected=off
  trigger_prediction : Outport  Port=3  VectorParamsAs1DForOutWhenUnconnected=off
  trigger_optimization : Outport  Port=4  VectorParamsAs1DForOutWhenUnconnected=off
  index : Outport  Port=5  VectorParamsAs1DForOutWhenUnconnected=off
  trigger_state_machine_finished : Outport  Port=6  VectorParamsAs1DForOutWhenUnconnected=off
  trigger_park_done_statemachine : Outport  Port=7  VectorParamsAs1DForOutWhenUnconnected=off
  wires:
  Delay9/1 -> trigger_voltages/1, Scope1/1
  OR/1 -> Delay9/1
  Switch5/1 -> index/1, Scope2/2, state_machine_flags/10, Scope1/3
  Delay8/1 -> Switch3/3
  Delay7/1 -> Switch3/1
  Switch3/1 -> Delay8/1, Switch5/3
  last_opt_index/1 -> Delay7/1
  Delay6/1 -> Switch2/3
  Delay5/1 -> Switch2/1
  AXI_no_of_iterations/1 -> Delay5/1
  Subsystem7/1(Q) -> Switch8/2  "Q"
  Subsystem7/2(!Q) -> Terminator7/1
  Switch8/1 -> OR/3  "Q"
  Delay4/1 -> Subsystem7/2(Reset), Subsystem2/2(Reset), state_machine_flags/9
  AND1/1 -> Delay4/1
  AND/1 -> trigger_state_machine_finished/1
  Switch9/1 -> trigger_prediction/1, Scope1/2
  Relational Operator1/1 -> AND/1, resetable_counter/2(rst), AND1/2
  resetable_counter/1(cnt) -> Relational Operator2/1, state_machine_flags/8, Scope/2
  Switch7/1 -> Switch/1
  Detect Rise Positive4/1 -> AND/2, state_machine_flags/5  "opt_done"
  HDL Counter/1 -> Relational Operator/1, state_machine_flags/6, Relational Operator1/1, Switch5/1  "index"
  Switch/1 -> HDL Counter/2
  Detect Rise Positive3/1 -> trigger_optimization/1, Scope2/1, Switch8/1, state_machine_flags/4, Switch7/1  "pred_done"
  limited_counter/1(cnt) -> Scope/1
  Relational Operator2/1 -> Subsystem2/1(Set)
  Constant4/1 -> limited_counter/1(limit), Relational Operator2/2
  Subsystem2/1(Q) -> Switch9/2, Switch7/2, state_machine_flags/7  "Q"
  Subsystem2/2(!Q) -> Terminator2/1
  Delay3/1 -> Detect Rise Positive1/1
  Detect Rise Positive1/1 -> Switch1/1, Switch9/1, AND1/1, state_machine_flags/2, limited_counter/2(enb), resetable_counter/1(enb)  "volts_done"
  Switch4/1 -> Subsystem/2(Reset), state_machine_flags/3  "delay_done"
  Detect Rise Positive2/1 -> Subsystem4/1(Set), Switch4/1, OR/2
  Subsystem4/2(!Q) -> Terminator4/1
  Subsystem4/1(Q) -> Switch4/2, Switch5/2  "Q"
  trigger_prediction_done/1 -> Delay1/1
  Delay1/1 -> Detect Rise Positive3/1
  trigger_optimization_done/1 -> Delay2/1
  Delay2/1 -> Detect Rise Positive4/1
  trigger_start_state_machine/1 -> Delay/1
  Delay/1 -> Detect Rise Positive/1
  Delay21/1 -> Detect Rise Positive2/1
  trigger_delay_comp_done/1 -> Delay21/1
  trigger_voltages_done/1 -> Delay3/1
  Switch1/1 -> trigger_delay_comp/1
  Subsystem/2(!Q) -> Terminator/1
  Subsystem/1(Q) -> Switch1/2  "Q"
  Detect Rise Positive/1 -> OR/1, trigger_park_done_statemachine/1, Subsystem4/2(Reset), Subsystem/1(Set), Subsystem7/1(Set), HDL Counter/1, state_machine_flags/1, Switch2/2, Switch3/2  "trigger_start"
  Relational Operator/1 -> Switch/2
  Switch2/1 -> Relational Operator1/2, Relational Operator/2, Delay6/1

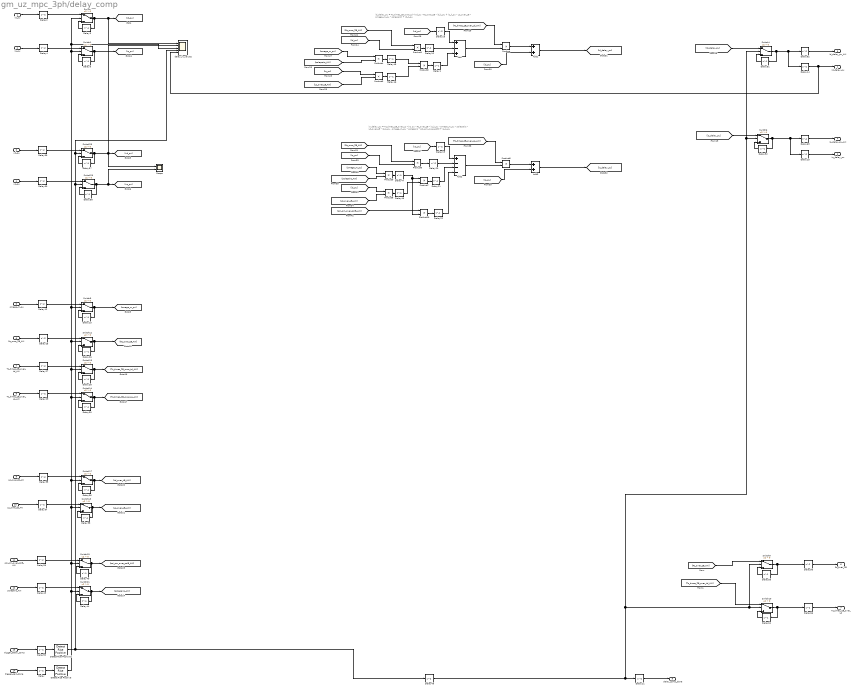
== system gm_uz_mpc_3ph/delay_comp ==
  note: id_delay_pu = Ts_times_ZB_over_Ld *(vd_pu - Rs_over_ZB * id_k_pu + iq_k_pu * Lq_over_LB * omega_m_pu * polepairs) + id_k_pu
  note: iq_delay_pu = Ts_times_ZB_over_Lq *(vq_pu - Rs_over_ZB * iq_k_pu - omega_m_pu * polepairs * Ld_over_LB * id_k_pu - omega_m_pu * polepairs * psi_pm_over_psiB) + iq_k_pu
  id_pu : Inport  OutDataTypeStr=fixdt_type_dq_currents
  iq_pu : Inport  Port=2  OutDataTypeStr=fixdt_type_dq_currents
  vd_pu : Inport  Port=3  OutDataTypeStr=fixdt_type_dqxy_voltages
  vq_pu : Inport  Port=4  OutDataTypeStr=fixdt_type_dqxy_voltages
  omega_m_pu : Inport  Port=5  OutDataTypeStr=fixdt_type_speed
  Rs_over_ZB_AXI : Inport  Port=6  OutDataTypeStr=fixdt_type_constants
  Ts_times_ZB_over_Ld_AXI : Inport  Port=7  OutDataTypeStr=fixdt_type_constants
  Ts_times_ZB_over_Lq_AXI : Inport  Port=8  OutDataTypeStr=fixdt_type_constants
  Ld_over_LB_AXI : Inport  Port=9  OutDataTypeStr=fixdt_type_constants
  Lq_over_LB_AXI : Inport  Port=10  OutDataTypeStr=fixdt_type_constants
  psi_pm_over_psiB_AXI : Inport  Port=11  OutDataTypeStr=fixdt_type_constants
  polepairs_AXI : Inport  Port=12  OutDataTypeStr=fixdt_type_polepairs
  trigger_delay_comp : Inport  Port=13
  trigger_park_done : Inport  Port=14
  Add : Sum  Inputs=+-+  AccumDataTypeStr=fixdt(1,27,16)
  Add1 : Sum  AccumDataTypeStr=fixdt(1,27,24)
  Add2 : Sum  Inputs=+---  AccumDataTypeStr=fixdt(1,27,16)
  Add3 : Sum  AccumDataTypeStr=fixdt(1,27,24)
  Delay{,2,4,10..12,14..15,18..20,25,27,29,35,37,39,43,49..50,56,59..60,62..63,66} (26 alike) : Delay
  Delay{1,3,5,13,21..22,26,28,30,36,38,40,44..48,51..52,55,57..58,61} (23 alike) : Delay  DelayLength=1
  Detect Rise Positive : simulink/Logic and Bit Operations/Detect Rise Positive  vinit=0  OutDataTypeStr=boolean
  Detect Rise Positive1 : simulink/Logic and Bit Operations/Detect Rise Positive  vinit=0  OutDataTypeStr=boolean
  Product{,1..2,4..7,9..10} (9 alike) : Product  OutDataTypeStr=fixdt(1,18,15)
  Product3 : Product  OutDataTypeStr=fixdt(1,27,16)
  Product8 : Product  OutDataTypeStr=fixdt(1,27,16)
  Scope : Scope  NumInputPorts=2
  Switch : Switch  Criteria=u2 > Threshold  OutDataTypeStr=fixdt_type_dq_currents
  Switch1 : Switch  Criteria=u2 > Threshold  OutDataTypeStr=fixdt_type_dq_currents
  Switch{4,6,9..10} (4 alike) : Switch  Criteria=u2 > Threshold
  Switch{12..14,17..19} (6 alike) : Switch  Criteria=u2 > Threshold  OutDataTypeStr=fixdt_type_constants
  Switch21 : Switch  Criteria=u2 > Threshold  OutDataTypeStr=fixdt_type_polepairs
  Switch28 : Switch  Criteria=u2 > Threshold  OutDataTypeStr=fixdt_type_dqxy_voltages
  Switch29 : Switch  Criteria=u2 > Threshold  OutDataTypeStr=fixdt_type_dqxy_voltages
  Switch5 : Switch  Criteria=u2 > Threshold  OutDataTypeStr=fixdt_type_speed
  delay_in_values : Scope  NumInputPorts=5
  id_delay_pu : Outport
  iq_delay_pu : Outport  Port=2
  id_delay_pu_AXI : Outport  Port=3
  iq_delay_pu_AXI : Outport  Port=4
  delay_comp_done : Outport  Port=5
  Rs_over_ZB : Outport  Port=6
  Ts_times_ZB_over_Ld : Outport  Port=7
  wires:
  Delay66/1 -> Ts_times_ZB_over_Ld/1
  [Ts_times_ZB_over_Ld_AXI] -> Switch10/1
  Delay61/1 -> Switch10/3
  Switch10/1 -> Delay66/1, Delay61/1
  Delay56/1 -> Rs_over_ZB/1
  Delay49/1 -> Delay11/1, Switch4/2, Switch6/2, Switch10/2, Switch9/2
  [Rs_over_ZB_AXI] -> Switch9/1
  Delay55/1 -> Switch9/3
  Switch9/1 -> Delay56/1, Delay55/1
  Delay52/1 -> Switch6/3
  Switch6/1 -> Delay63/1, Delay15/1, Delay52/1
  [iq_delay_pu] -> Switch6/1
  Delay51/1 -> Switch4/3
  [id_delay_pu] -> Switch4/1
  Detect Rise Positive1/1 -> Switch29/2, Switch28/2, delay_in_values/4, Delay49/1  "delay_comp done"
  Detect Rise Positive/1 -> delay_in_values/3, Switch/2, Switch1/2, Switch5/2, Switch12/2, Switch13/2, Switch14/2, Switch17/2, Switch18/2, Switch19/2, Switch21/2
  Delay50/1 -> Detect Rise Positive1/1
  trigger_delay_comp/1 -> Delay50/1
  Delay48/1 -> Product7/2
  Product8/1 -> Delay48/1
  Delay47/1 -> Product7/1, Product10/2
  Product9/1 -> Delay47/1
  Delay45/1 -> Product2/1
  Delay46/1 -> Product2/2
  Product3/1 -> Delay46/1
  Product4/1 -> Delay45/1
  Product6/1 -> Delay20/1
  Delay19/1 -> Add2/1
  Delay20/1 -> Add2/2
  Delay21/1 -> Add2/3
  Delay22/1 -> Add2/4
  Product10/1 -> Delay22/1
  Product7/1 -> Delay21/1
  [vq_pu] -> Delay19/1  "vq_pu"
  Delay18/1 -> Add/1
  [vd_pu] -> Delay18/1  "vd_pu"
  Delay1/1 -> Add/3
  Delay10/1 -> Add/2
  Product1/1 -> Delay10/1
  Product2/1 -> Delay1/1
  [psi_pm_over_psiB_AXI] -> Product10/1
  Product5/1 -> Add3/1
  [polepairs_AXI] -> Product9/2  "polepairs"
  [Ld_over_LB_AXI] -> Product8/2  "Ld_over_LB"
  [id_pu] -> Product8/1  "id_k_pu"
  [iq_pu] -> Add3/2  "iq_k_pu"
  [omega_m_pu] -> Product9/1  "omega_m_pu"
  Add2/1 -> Product5/2
  [Rs_over_ZB_AXI] -> Product6/1  "Rs_over_ZB"
  [iq_pu] -> Product6/2  "iq_k_pu"
  [Ts_times_ZB_over_Lq_AXI] -> Product5/1  "Ts_times_ZB_over_Lq"
  [polepairs_AXI] -> Product4/2  "polepairs"
  [omega_m_pu] -> Product4/1  "omega_m_pu"
  [Lq_over_LB_AXI] -> Product3/2  "Lq_over_LB"
  [iq_pu] -> Product3/1  "iq_k_pu"
  [id_pu] -> Product1/2  "id_k_pu"
  [Rs_over_ZB_AXI] -> Product1/1  "Rs_over_ZB"
  [id_pu] -> Add1/2  "id_k_pu"
  Product/1 -> Add1/1
  [Ts_times_ZB_over_Ld_AXI] -> Product/1  "Ts_times_ZB_over_Ld"
  Add/1 -> Product/2
  Delay14/1 -> id_delay_pu/1, delay_in_values/5
  Delay15/1 -> iq_delay_pu/1
  Delay62/1 -> id_delay_pu_AXI/1
  Delay63/1 -> iq_delay_pu_AXI/1
  Switch4/1 -> Delay62/1, Delay14/1, Delay51/1
  Delay11/1 -> delay_comp_done/1
  Delay30/1 -> Switch14/3
  Delay36/1 -> Switch17/3
  Delay13/1 -> Switch5/3
  Delay40/1 -> Switch19/3
  trigger_park_done/1 -> Delay/1
  Delay39/1 -> Switch19/1
  Rs_over_ZB_AXI/1 -> Delay25/1
  Delay57/1 -> Switch28/3
  Ts_times_ZB_over_Ld_AXI/1 -> Delay27/1
  Switch1/1 -> Delay5/1, [iq_pu]
  Switch19/1 -> Delay40/1, [psi_pm_over_psiB_AXI]
  Delay26/1 -> Switch12/3
  Switch18/1 -> [Lq_over_LB_AXI], Delay38/1
  Delay3/1 -> Switch/3
  Ts_times_ZB_over_Lq_AXI/1 -> Delay29/1
  Delay60/1 -> Switch29/1
  iq_pu/1 -> Delay4/1
  Lq_over_LB_AXI/1 -> Delay37/1
  Switch5/1 -> Delay13/1, [omega_m_pu]
  vq_pu/1 -> Delay60/1
  Delay27/1 -> Switch13/1
  omega_m_pu/1 -> Delay12/1
  Delay12/1 -> Switch5/1
  Delay4/1 -> Switch1/1
  Delay37/1 -> Switch18/1
  Switch28/1 -> Delay57/1, [vd_pu], delay_in_values/2, Scope/1
  Delay35/1 -> Switch17/1
  Switch/1 -> Delay3/1, [id_pu], delay_in_values/1
  Switch21/1 -> Delay44/1, [polepairs_AXI]
  id_pu/1 -> Delay2/1
  Delay58/1 -> Switch29/3
  psi_pm_over_psiB_AXI/1 -> Delay39/1
  Delay28/1 -> Switch13/3
  Switch14/1 -> Delay30/1, [Ts_times_ZB_over_Lq_AXI]
  Delay43/1 -> Switch21/1
  polepairs_AXI/1 -> Delay43/1
  Switch29/1 -> Delay58/1, [vq_pu], Scope/2
  Delay29/1 -> Switch14/1
  Delay44/1 -> Switch21/3
  Delay/1 -> Detect Rise Positive/1
  Switch13/1 -> Delay28/1, [Ts_times_ZB_over_Ld_AXI]
  Switch17/1 -> [Ld_over_LB_AXI], Delay36/1
  Delay38/1 -> Switch18/3
  Delay2/1 -> Switch/1
  Ld_over_LB_AXI/1 -> Delay35/1
  vd_pu/1 -> Delay59/1
  Delay59/1 -> Switch28/1
  Delay25/1 -> Switch12/1
  Delay5/1 -> Switch1/3
  Add1/1 -> [id_delay_pu]
  Add3/1 -> [iq_delay_pu]
  Switch12/1 -> Delay26/1, [Rs_over_ZB_AXI]
